simulink model "dac"  (R2016b)
settings: Solver=VariableStepAuto  StartTime=0.0  StopTime=0.01  MaxStep=0.2  RelTol=1e-3
libraries: simulink x1
settings Model: Creator=jeff  LastModifiedBy=jeff

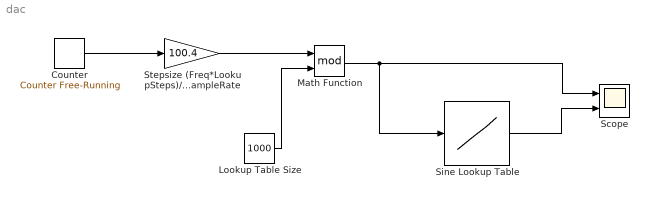
== system dac ==
  Counter : simulink/Sources/Counter Free-Running  NumBits=16  tsamp=0.0001
  Lookup Table Size : Constant  Value=1000  OutDataTypeStr=int32
  Math Function : Math  Operator=mod  SaturateOnIntegerOverflow=on
  Scope : Scope  NumInputPorts=2
  Sine Lookup Table : Lookup_n-D  NumberOfTableDimensions=1  BreakpointsSpecification=Even spacing  BreakpointsForDimension1=[0:7]  BreakpointsForDimension1FirstPoint=0  Table=(2^15) * sin(2*pi*[0:1000]/1000)  InterpMethod=Flat  InternalRulePriority=Speed  OutDataTypeStr=int16  RndMeth=Simplest  InputSameDT=on
  Stepsize (Freq*LookupSteps)/SampleRate : Gain  Gain=100.4  OutDataTypeStr=int32
  wires:
  Sine Lookup Table/1 -> Scope/2
  Counter/1 -> Stepsize (Freq*LookupSteps)/SampleRate/1
  Stepsize (Freq*LookupSteps)/SampleRate/1 -> Math Function/1
  Math Function/1 -> Scope/1, Sine Lookup Table/1
  Lookup Table Size/1 -> Math Function/2
